simulink model "pulseshaping"  (R2020b)
settings: Solver=VariableStepAuto  StartTime=0.0  StopTime=600e-6  RelTol=1e-3
values from neighbouring files (symbols this model uses):
  a_fir_coeff = [     a_filter_slope_pos  .* ones(1,a_filter_slope_length),                           zeros(1,a_filter_gap_length),      a_filter_slope_neg  .* ones(1,a_filter_slope_length)   ]    [file_pulse_shaping_params.m]    (also in pulse_shaping_params.m)
  hpf_diff_constant = 140e-9    (= 1.4e-07)    [file_pulse_shaping_params.m]    (also in pulse_shaping_params.m = 5e-05)
  lp_coeff = ones(1,ma_length)./ma_length    [file_pulse_shaping_params.m]    (also in pulse_shaping_params.m)
  nakhostin_10_1_eneg = exp(-sampling_rate/2/hpf_diff_constant)    [file_pulse_shaping_params.m]    (also in pulse_shaping_params.m)
  nakhostin_10_1_epos = exp(sampling_rate/2/hpf_diff_constant)    [file_pulse_shaping_params.m]    (also in pulse_shaping_params.m)
  nakhostin_10_1_L = 30    [file_pulse_shaping_params.m]    (also in pulse_shaping_params.m = 16)
  nakhostin_10_3_fir_coeff = [0,ones(1,nakhostin_10_3_L-1)]    [file_pulse_shaping_params.m]    (also in pulse_shaping_params.m)
  nakhostin_10_3_gain = sampling_rate/2/hpf_diff_constant    (= 0.00357142857143)    [file_pulse_shaping_params.m]    (also in pulse_shaping_params.m = 0.001)
  nakhostin_10_3_L = 48    [file_pulse_shaping_params.m]    (also in pulse_shaping_params.m = 8)
  pulse_gen_noise_clock = 50e-9    (= 5e-08)    [file_pulse_shaping_params.m]    (also in pulse_shaping_params.m = 2e-05)
  pulse_gen_period = 1*1e-8    (= 1e-08)    [file_pulse_shaping_params.m]    (also in pulse_shaping_params.m = 0.0001)
  sampling_rate = 1e-9    (= 1e-09)    [file_pulse_shaping_params.m]    (also in pulse_shaping_params.m = 1e-07)
libraries: dspstat3 x3, simulink x2
settings Model: Creator=Dickbutt  LastModifiedBy=Dickbutt

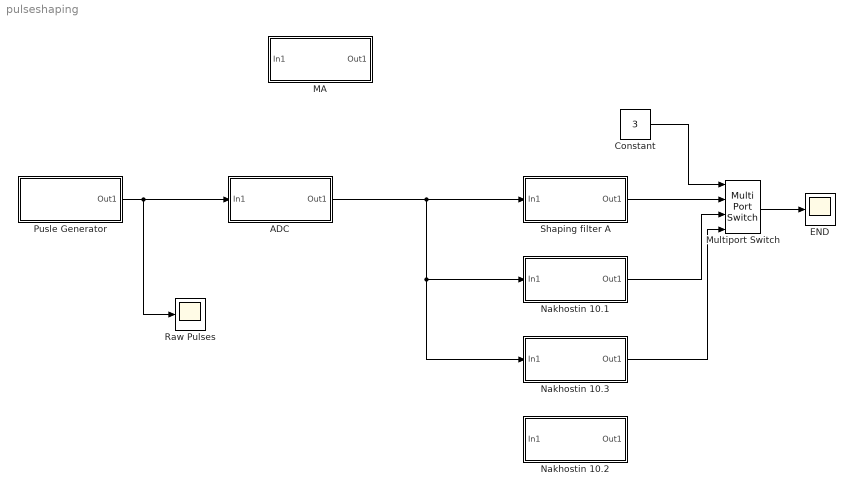
== system pulseshaping ==
  ADC : Subsystem
  Constant : Constant  Value=3
  END : Scope
  MA : Subsystem
  Multiport Switch : MultiPortSwitch
  Nakhostin 10.1 : Subsystem
  Nakhostin 10.2 : Subsystem
  Nakhostin 10.3 : Subsystem
  Pusle Generator : Subsystem
  Raw Pulses : Scope
  Shaping filter A : Subsystem
  wires:
  Multiport Switch/1 -> END/1
  Nakhostin 10.1/1(Out1) -> Multiport Switch/3
  Shaping filter A/1(Out1) -> Multiport Switch/2
  Constant/1 -> Multiport Switch/1
  Nakhostin 10.3/1(Out1) -> Multiport Switch/4
  Pusle Generator/1(Out1) -> ADC/1(In1), Raw Pulses/1
  ADC/1(Out1) -> Nakhostin 10.3/1(In1), Nakhostin 10.1/1(In1), Shaping filter A/1(In1)

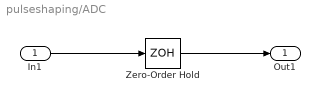
== system pulseshaping/ADC ==
  In1 : Inport
  Zero-Order Hold : ZeroOrderHold  SampleTime=sampling_rate
  Out1 : Outport
  wires:
  In1/1 -> Zero-Order Hold/1
  Zero-Order Hold/1 -> Out1/1

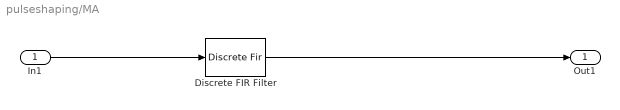
== system pulseshaping/MA ==
  In1 : Inport
  Discrete FIR Filter : DiscreteFir  Coefficients=lp_coeff
  Out1 : Outport
  wires:
  In1/1 -> Discrete FIR Filter/1
  Discrete FIR Filter/1 -> Out1/1

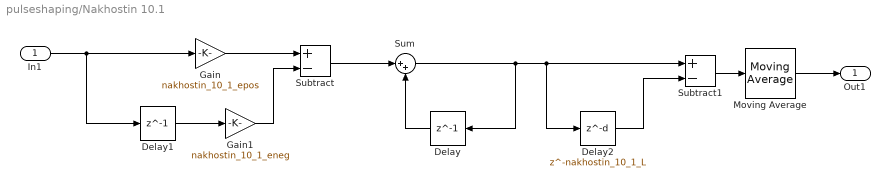
== system pulseshaping/Nakhostin 10.1 ==
  In1 : Inport
  Delay : Delay  DelayLength=1  InitialCondition=0
  Delay1 : Delay  DelayLength=1  InitialCondition=0
  Delay2 : Delay  DelayLength=nakhostin_10_1_L  InitialCondition=0
  Gain : Gain  Gain=nakhostin_10_1_epos
  Gain1 : Gain  Gain=nakhostin_10_1_eneg
  Moving Average : dspstat3/Moving Average  Method=Sliding window  ForgettingFactorPort=off  SpecifyWindowLength=on  WindowLength=nakhostin_10_1_MA_order  ForgettingFactor=0.9  SimulateUsing=Code generation
  Subtract : Sum  Inputs=+-
  Subtract1 : Sum  Inputs=+-
  Sum : Sum  Inputs=|++
  Out1 : Outport
  wires:
  Delay1/1 -> Gain1/1
  Gain1/1 -> Subtract/2
  Gain/1 -> Subtract/1
  Delay/1 -> Sum/2
  In1/1 -> Delay1/1, Gain/1
  Subtract/1 -> Sum/1
  Sum/1 -> Delay2/1, Subtract1/1, Delay/1
  Delay2/1 -> Subtract1/2
  Subtract1/1 -> Moving Average/1
  Moving Average/1 -> Out1/1

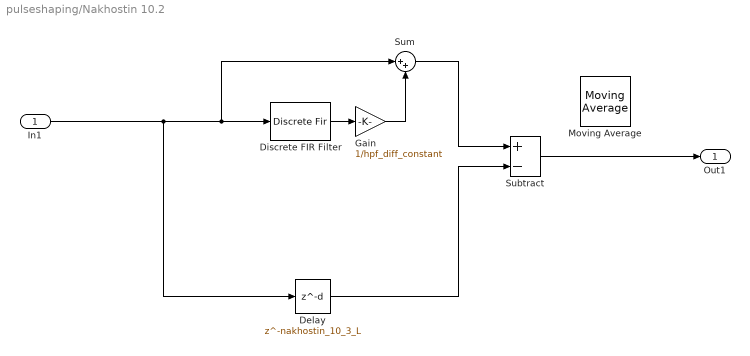
== system pulseshaping/Nakhostin 10.2 ==
  In1 : Inport
  Delay : Delay  DelayLength=nakhostin_10_3_L  InitialCondition=0
  Discrete FIR Filter : DiscreteFir  Coefficients=nakhostin_10_3_fir_coeff
  Gain : Gain  Gain=1/hpf_diff_constant
  Moving Average : dspstat3/Moving Average  Method=Sliding window  ForgettingFactorPort=off  SpecifyWindowLength=on  WindowLength=nakhostin_10_3_N  ForgettingFactor=0.9  SimulateUsing=Code generation
  Subtract : Sum  Inputs=+-
  Sum : Sum  Inputs=|++
  Out1 : Outport
  wires:
  In1/1 -> Delay/1, Discrete FIR Filter/1, Sum/1
  Discrete FIR Filter/1 -> Gain/1
  Gain/1 -> Sum/2
  Sum/1 -> Subtract/1
  Delay/1 -> Subtract/2
  Subtract/1 -> Out1/1

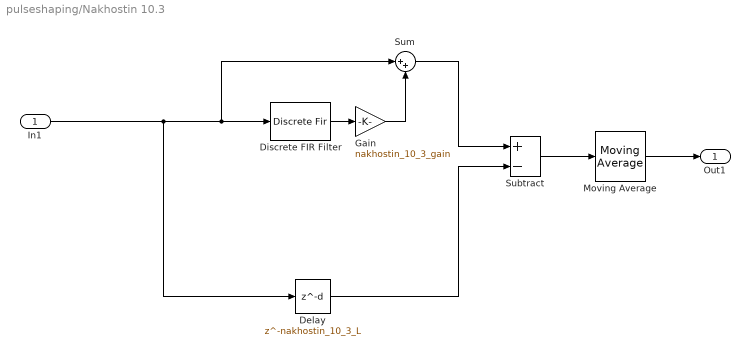
== system pulseshaping/Nakhostin 10.3 ==
  In1 : Inport
  Delay : Delay  DelayLength=nakhostin_10_3_L  InitialCondition=0
  Discrete FIR Filter : DiscreteFir  Coefficients=nakhostin_10_3_fir_coeff
  Gain : Gain  Gain=nakhostin_10_3_gain
  Moving Average : dspstat3/Moving Average  Method=Sliding window  ForgettingFactorPort=off  SpecifyWindowLength=on  WindowLength=nakhostin_10_3_N  ForgettingFactor=0.9  SimulateUsing=Code generation
  Subtract : Sum  Inputs=+-
  Sum : Sum  Inputs=|++
  Out1 : Outport
  wires:
  In1/1 -> Delay/1, Discrete FIR Filter/1, Sum/1
  Discrete FIR Filter/1 -> Gain/1
  Gain/1 -> Sum/2
  Sum/1 -> Subtract/1
  Delay/1 -> Subtract/2
  Subtract/1 -> Moving Average/1
  Moving Average/1 -> Out1/1

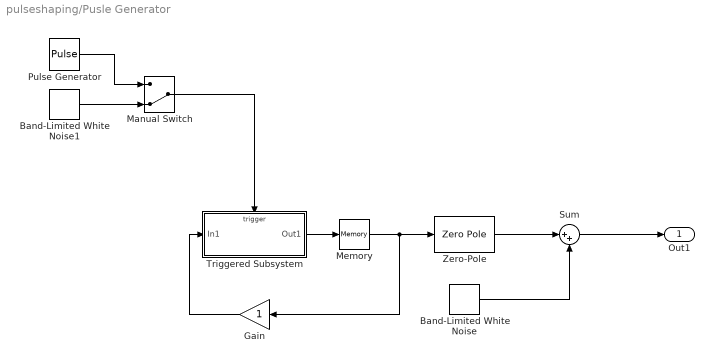
== system pulseshaping/Pusle Generator ==
  Band-Limited White Noise : simulink/Sources/Band-Limited White Noise  Cov=noise_power  Ts=sampling_rate  seed=[23341]
  Band-Limited White Noise1 : simulink/Sources/Band-Limited White Noise  Cov=[0.5]  Ts=pulse_gen_noise_clock  seed=[23341]
  Gain : Gain
  Manual Switch : ManualSwitch  CurrentSetting=0
  Memory : Memory
  Pulse Generator : DiscretePulseGenerator  PulseType=Time based  Period=pulse_gen_period  PulseWidth=5
  Sum : Sum  Inputs=|++
  Triggered Subsystem : Subsystem  TreatAsAtomicUnit=on
  Zero-Pole : ZeroPole  Zeros=[0]  Poles=[-1/hpf_diff_constant]  Gain=[0.8]
  Out1 : Outport
  wires:
  Pulse Generator/1 -> Manual Switch/1
  Triggered Subsystem/1(Out1) -> Memory/1
  Memory/1 -> Zero-Pole/1, Gain/1
  Gain/1 -> Triggered Subsystem/1(In1)
  Zero-Pole/1 -> Sum/1
  Band-Limited White Noise/1 -> Sum/2
  Sum/1 -> Out1/1
  Band-Limited White Noise1/1 -> Manual Switch/2
  Manual Switch/1 -> Triggered Subsystem/Trigger

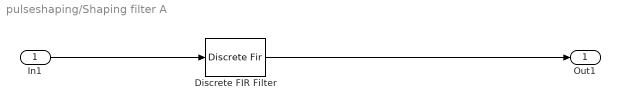
== system pulseshaping/Shaping filter A ==
  In1 : Inport
  Discrete FIR Filter : DiscreteFir  Coefficients=a_fir_coeff
  Out1 : Outport
  wires:
  In1/1 -> Discrete FIR Filter/1
  Discrete FIR Filter/1 -> Out1/1

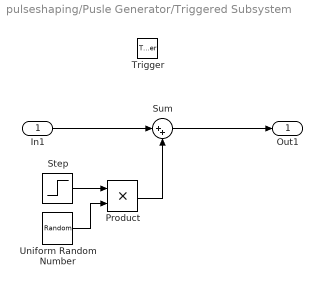
== system pulseshaping/Pusle Generator/Triggered Subsystem ==
  In1 : Inport
  Trigger : TriggerPort  VariantControl=Variant
  Product : Product
  Step : Step  Time=0
  Sum : Sum  Inputs=|++
  Uniform Random Number : UniformRandomNumber  Minimum=0.1  Maximum=2  Seed=rand(1)
  Out1 : Outport
  wires:
  In1/1 -> Sum/1
  Sum/1 -> Out1/1
  Step/1 -> Product/1
  Uniform Random Number/1 -> Product/2
  Product/1 -> Sum/2
